simulink library "myLibrary"  (R2023a)
settings: Solver=VariableStepAuto  StartTime=0.0  StopTime=10.0  RelTol=1e-3
undefined symbols (not defined in the file): Cac_n1, ctrl1, Da, Discrete, dtha, ee_sli_rtmsupport, FA, gcbh, Ha, Ini, init_line, init_load, init_SG, init_TH, init_trafo, init_VSC, initMachineBlocks, Ka, Lf, Llkd_pu, Llkq1_pu, NET, P, plots_step, q0, Rac_n1, Radd, Rkd_pu, Rkq1_pu, Rload_add, sim_config, spsSteamTurbineModel, T_global, T_load, T_NET, T_SG, T_TH, T_trafo, T_VSC, Ts, tstep, V1
libraries: spsSeriesRLCBranchLib x57, spsParallelRLCBranchLib x39, eeGeneralControl x38, spsCurrentMeasurementLib x20, spsFirstOrderFilterLib x16, spsVoltageMeasurementLib x14, spsControlledVoltageSourceLib x12, $bdroot x9, dspsigops x6, spsThreePhaseVIMeasurementLib x5, spsPLL3phLib x4, spsThreePhaseBreakerLib x3
(part 2 of 7)

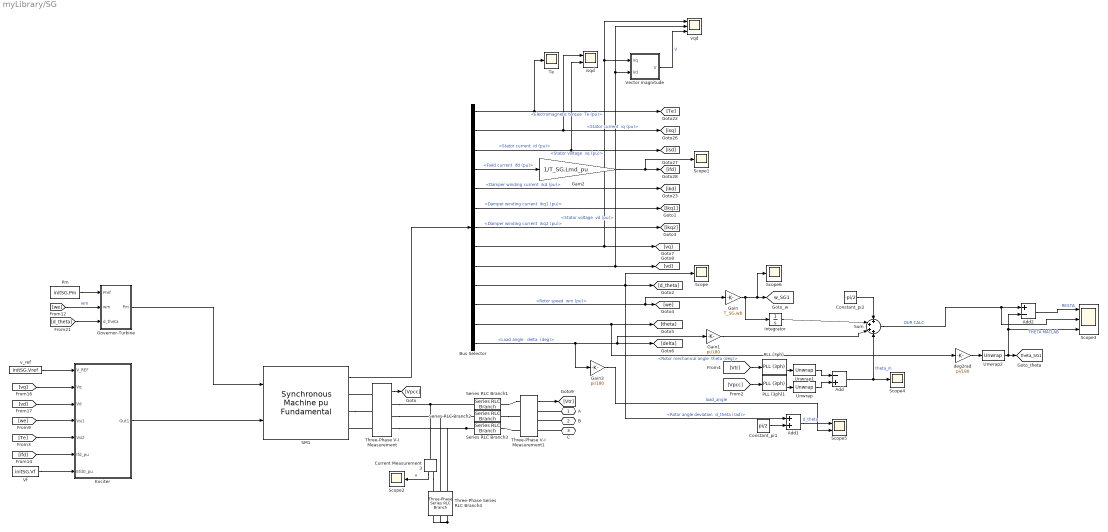
== system myLibrary/SG ==
  Add : Sum  Inputs=-+
  Add1 : Sum
  Add2 : Sum  Inputs=+-
  Bus Selector : BusSelector  OutputSignals="Mechanical.Electromagnetic torque  Te (pu),dq0 components.Stator current  iq (pu),dq0 components.Stator current  id (pu),dq0 components.Field current  ifd (pu),dq0 components.Damper winding current  ikd (pu),dq0 components.Damper winding current  ikq1 (pu),dq0 components.Damper winding current  ikq2 (pu),dq0 components.Stator voltage  vq (pu),dq0 components.Stator voltage  vd (pu),Mechanical.Rotor angle deviation  d_theta (rad),Mechanical.Rotor speed  wm (pu),Mechanical.Rotor mechanical angle  theta (deg),Load angle   delta  (deg)"
  Constant_pi1 : Constant  Value=pi/2
  Constant_pi2 : Constant  Value=-pi/2
  Current Measurement3 : spsCurrentMeasurementLib/Current Measurement  PhasorSimulation=off  OutputType=Complex  PSBequivalent=0
  Exciter : Subsystem
  Gain : Gain  Gain=T_SG.wb
  Gain1 : Gain  Gain=pi/180
  Gain2 : Gain  Gain=1/T_SG.Lmd_pu
  Gain3 : Gain  Gain=pi/180
  Governor-Turbine : Subsystem
  Integrator : Integrator
  PLL (3ph) : spsPLL3phLib/PLL (3ph)  Fmin=45  Par_Init=[0, 50]  ParK=[180, 3200, 1]  TcD=1e-4  MaxRateChangeFreq=12  FilterCutOffFreq=25  Ts=0  AGC=on
  PLL (3ph)1 : spsPLL3phLib/PLL (3ph)  Fmin=45  Par_Init=[initSG.theta_in, 50]  ParK=[180, 3200, 1]  TcD=1e-4  MaxRateChangeFreq=12  FilterCutOffFreq=25  Ts=0  AGC=on
  Pm : Constant  Value=initSG.Pm
  SM1 : spsSynchronousMachinepuFundamentalLib/Synchronous Machine pu Fundamental  PresetModel=No  MechanicalLoad=Mechanical power Pm  ShowDetailedParameters=on  RotorType=Round  Units=per unit fundamental parameters  MeasurementBus=off  NominalParameters=initMachineBlocks{SGnum,1}  Stator=initMachineBlocks{SGnum,2}  Field=initMachineBlocks{SGnum,3}  Dampers2=initMachineBlocks{SGnum,4}  Dampers1="[ Rkd_pu   Llkd_pu  Rkq1_pu  Llkq1_pu]"  Mechanical=initMachineBlocks{SGnum,5}  PolePairs=1  InitialConditions=initMachineBlocks{SGnum,6}  SetSaturation=off  Saturation=[0.6404,0.7127,0.8441,0.9214,0.9956,1.082,1.19,1.316,1.457;0.7,0.7698,0.8872,0.9466,0.9969,1.046,1.1,1.151,1.201]  LoadFlowParameters=[1 5.55 0 0 0]  TsPowergui=0  TsBlock=-1  IterativeModel=Trapezoidal non iterative  IterativeDiscreteModel=Trapezoidal non iterative  BusType=PV  Pref=5.55  Qref=0  Qmin=-Inf  Qmax=Inf  PLF=0  QLF=0
  Scope{,1..2,4,6} (5 alike) : Scope
  Scope3 : Scope  NumInputPorts=3
  Scope5 : Scope  NumInputPorts=2
  Series RLC Branch1 : spsSeriesRLCBranchLib/Series RLC Branch  LConnTagsString=__new0  RConnTagsString=__new0  BranchType=RL  Resistance=T_SG.Rtr*T_SG.Zbpu_l2g  Inductance=T_SG.Ltr*T_SG.Zbpu_l2g  SetiL0=off  InitialCurrent=initSG.Itr  Capacitance=P.C  Setx0=on  InitialVoltage=P.C  Measurements=None
  Series RLC Branch2 : spsSeriesRLCBranchLib/Series RLC Branch  LConnTagsString=__new0  RConnTagsString=__new0  BranchType=RL  Resistance=T_SG.Rtr*T_global.Sb(T_global.Area == T_SG.Area)/T_SG.Sb  Inductance=T_SG.Ltr*T_global.Sb(T_global.Area == T_SG.Area)/T_SG.Sb  SetiL0=off  InitialCurrent=initSG.Itr  Capacitance=P.C  Setx0=on  InitialVoltage=P.C  Measurements=None
  Series RLC Branch3 : spsSeriesRLCBranchLib/Series RLC Branch  LConnTagsString=__new0  RConnTagsString=__new0  BranchType=RL  Resistance=T_SG.Rtr*T_global.Sb(T_global.Area == T_SG.Area)/T_SG.Sb  Inductance=T_SG.Ltr*T_global.Sb(T_global.Area == T_SG.Area)/T_SG.Sb  SetiL0=off  InitialCurrent=initSG.Itr  Capacitance=P.C  Setx0=on  InitialVoltage=P.C  Measurements=None
  Sum : Sum  Inputs=++++
  Te : Scope
  Three-Phase Series RLC Branch4 : spsThreePhaseSeriesRLCBranchLib/Three-Phase Series RLC Branch  LConnTagsString=A|B|C  RConnTagsString=A|B|C  BranchType=R  Resistance=T_SG.Rsnb*T_SG.Zbpu_l2g  Inductance=NET.L1_2/2  Capacitance=1/0.0528/(2*pi*50)  Measurements=None
  Three-Phase V-I Measurement : spsThreePhaseVIMeasurementLib/Three-Phase V-I Measurement  VoltageMeasurement=phase-to-phase  SetLabelV=off  LabelV=Vpcc  Vpu=off  VpuLL=off  CurrentMeasurement=no  SetLabelI=off  LabelI=Iabc  Ipu=off  Pbase=100e6  Vbase=500e3  OutputType=Complex  PhasorSimulation=off  PSBequivalent=0
  Three-Phase V-I Measurement1 : spsThreePhaseVIMeasurementLib/Three-Phase V-I Measurement  VoltageMeasurement=phase-to-phase  SetLabelV=off  LabelV=Vtr  Vpu=off  VpuLL=off  CurrentMeasurement=no  SetLabelI=off  LabelI=Iabc  Ipu=off  Pbase=100e6  Vbase=500e3  OutputType=Complex  PhasorSimulation=off  PSBequivalent=0
  Unwrap : dspsigops/Unwrap  tol=pi  InputProcessing=Columns as channels (frame based)  running=off
  Unwrap1 : dspsigops/Unwrap  tol=pi  InputProcessing=Columns as channels (frame based)  running=off
  Unwrap2 : dspsigops/Unwrap  tol=pi  InputProcessing=Columns as channels (frame based)  running=off
  "Vector magnitude " : Subsystem
  Vf : Constant  Value=initSG.Vf
  deg2rad : Gain  Gain=pi/180
  isqd : Scope  NumInputPorts=2
  v_ref : Constant  Value=initSG.Vref
  vqd : Scope  NumInputPorts=3
  A : PMIOPort  Side=Right
  B : PMIOPort  Port=2  Side=Right
  C : PMIOPort  Port=3  Side=Right
  tag scope: theta_SG1=global, w_SG1=global
  wires:
  Three-Phase V-I Measurement1/1 -> [Vtr]
  Three-Phase V-I Measurement/1 -> [Vpcc]
  Bus Selector/10 -> [d_theta], Add1/1, Scope/1  "<Rotor angle deviation  d_theta (rad)>"
  Bus Selector/7 -> [ikq2]  "<Damper winding current  ikq2 (pu)>"
  [Vtr] -> PLL (3ph)/1
  Gain2/1 -> Scope1/1, [ifd]
  Bus Selector/5 -> [ikd]  "<Damper winding current  ikd (pu)>"
  Bus Selector/3 -> isqd/2, [isd]  "<Stator current  id (pu)>"
  Bus Selector/11 -> [we], Gain/1  "<Rotor speed  wm (pu)>"
  Bus Selector/6 -> [ikq1]  "<Damper winding current  ikq1 (pu)>"
  [Vpcc] -> PLL (3ph)1/1
  Bus Selector/4 -> Gain2/1  "<Field current  ifd (pu)>"
  Bus Selector/8 -> "Vector magnitude "/1(Vq), vqd/1, [vq]  "<Stator voltage  vq (pu)>"
  Bus Selector/1 -> Te/1, [Te]  "<Electromagnetic torque  Te (pu)>"
  Bus Selector/9 -> "Vector magnitude "/2(Vd), vqd/2, [vd]  "<Stator voltage  vd (pu)>"
  Gain/1 -> Scope6/1, [w_SG1], Integrator/1
  Current Measurement3/1 -> Scope2/1  "a"
  "Vector magnitude "/1(V) -> vqd/3  "V"
  Unwrap1/1 -> Add/1
  SM1/1 -> Bus Selector/1
  Bus Selector/13 -> [delta], Gain1/1, Gain3/1  "<Load angle   delta  (deg)>"
  Bus Selector/12 -> deg2rad/1, [theta]  "<Rotor mechanical angle  theta (deg)>"
  Bus Selector/2 -> isqd/1, [isq]  "<Stator current  iq (pu)>"
  Add/1 -> Scope4/1, Sum/4  "theta_in"
  Integrator/1 -> Sum/2
  PLL (3ph)1/2 -> Unwrap/1
  PLL (3ph)/2 -> Unwrap1/1
  Unwrap/1 -> Add/2
  Constant_pi1/1 -> Add1/2
  Add1/1 -> Scope5/1  "d_theta"
  Gain3/1 -> Scope5/2  "load_angle"
  Gain1/1 -> Sum/3
  Constant_pi2/1 -> Sum/1
  Governor-Turbine/1(Pm) -> SM1/1
  [we] -> Governor-Turbine/2(wm)  "wm"
  Pm/1 -> Governor-Turbine/1(Pref)
  [d_theta] -> Governor-Turbine/3(d_theta)
  deg2rad/1 -> Unwrap2/1
  Unwrap2/1 -> Add2/2, Scope3/3, [theta_SG1]  "THETA MATLAB"
  [we] -> Exciter/4(Vsi1)
  [vd] -> Exciter/3(Vd)
  [ifd] -> Exciter/6(Ifd_pu)
  [Te] -> Exciter/5(Vsi2)
  Vf/1 -> Exciter/7(Efd0_pu)
  v_ref/1 -> Exciter/1(V_REF)
  Exciter/1(Out1) -> SM1/2
  [vq] -> Exciter/2(Vq)
  Sum/1 -> Scope3/2, Add2/1  "OUR CALC"
  Add2/1 -> Scope3/1  "RESTA"
  connections:
  Three-Phase V-I Measurement/LConn3 -- SM1/RConn3
  SM1/RConn2 -- Three-Phase V-I Measurement/LConn2
  Three-Phase V-I Measurement/LConn1 -- SM1/RConn1
  B/RConn1 -- Three-Phase V-I Measurement1/RConn2
  Three-Phase V-I Measurement1/LConn3 -- Series RLC Branch3/RConn1
  Series RLC Branch1/RConn1 -- Three-Phase V-I Measurement1/LConn1
  Current Measurement3/RConn1 -- Three-Phase Series RLC Branch4/RConn1
  A/RConn1 -- Three-Phase V-I Measurement1/RConn1
  C/RConn1 -- Three-Phase V-I Measurement1/RConn3
  Series RLC Branch2/RConn1 -- Three-Phase V-I Measurement1/LConn2
  Three-Phase V-I Measurement/RConn1 -- Series RLC Branch1/LConn1 -- Current Measurement3/LConn1
  Series RLC Branch3/LConn1 -- Three-Phase V-I Measurement/RConn3 -- Three-Phase Series RLC Branch4/RConn3
  Three-Phase Series RLC Branch4/LConn3 -- Three-Phase Series RLC Branch4/LConn2 -- Three-Phase Series RLC Branch4/LConn1
  Series RLC Branch2/LConn1 -- Three-Phase V-I Measurement/RConn2 -- Three-Phase Series RLC Branch4/RConn2

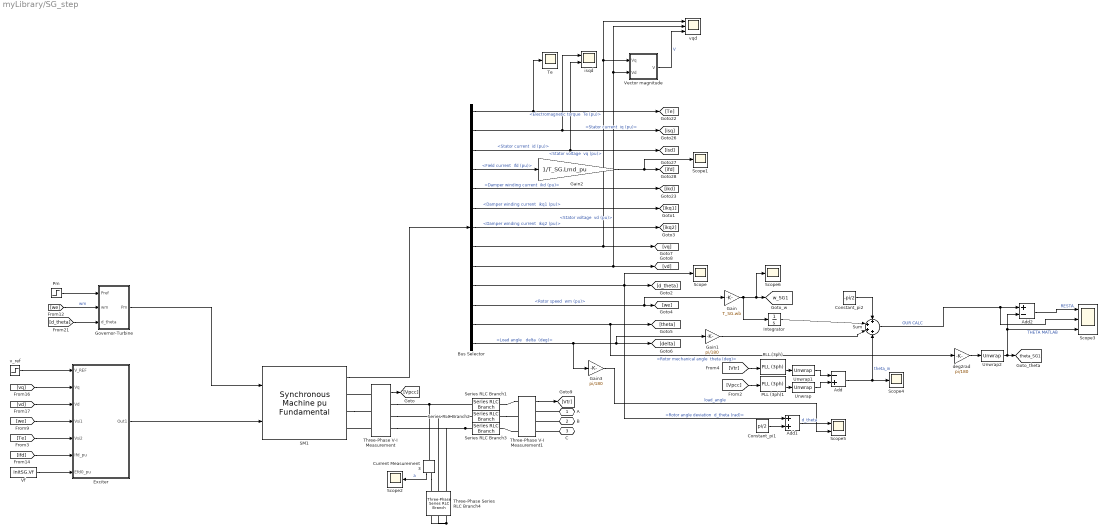
== system myLibrary/SG_step ==
  Add : Sum  Inputs=-+
  Add1 : Sum
  Add2 : Sum  Inputs=+-
  Bus Selector : BusSelector  OutputSignals="Mechanical.Electromagnetic torque  Te (pu),dq0 components.Stator current  iq (pu),dq0 components.Stator current  id (pu),dq0 components.Field current  ifd (pu),dq0 components.Damper winding current  ikd (pu),dq0 components.Damper winding current  ikq1 (pu),dq0 components.Damper winding current  ikq2 (pu),dq0 components.Stator voltage  vq (pu),dq0 components.Stator voltage  vd (pu),Mechanical.Rotor angle deviation  d_theta (rad),Mechanical.Rotor speed  wm (pu),Mechanical.Rotor mechanical angle  theta (deg),Load angle   delta  (deg)"
  Constant_pi1 : Constant  Value=pi/2
  Constant_pi2 : Constant  Value=-pi/2
  Current Measurement3 : spsCurrentMeasurementLib/Current Measurement  PhasorSimulation=off  OutputType=Complex  PSBequivalent=0
  Exciter : Subsystem
  Gain : Gain  Gain=T_SG.wb
  Gain1 : Gain  Gain=pi/180
  Gain2 : Gain  Gain=1/T_SG.Lmd_pu
  Gain3 : Gain  Gain=pi/180
  Governor-Turbine : Subsystem
  Integrator : Integrator
  PLL (3ph) : spsPLL3phLib/PLL (3ph)  Fmin=45  Par_Init=[0, 50]  ParK=[180, 3200, 1]  TcD=1e-4  MaxRateChangeFreq=12  FilterCutOffFreq=25  Ts=0  AGC=on
  PLL (3ph)1 : spsPLL3phLib/PLL (3ph)  Fmin=45  Par_Init=[initSG.theta_in, 50]  ParK=[180, 3200, 1]  TcD=1e-4  MaxRateChangeFreq=12  FilterCutOffFreq=25  Ts=0  AGC=on
  Pm : Step  Time=tstep_P  Before=initSG.Pm  After=initSG.Pm*(1+sim_config.DR)  SampleTime=1e-4
  SM1 : spsSynchronousMachinepuFundamentalLib/Synchronous Machine pu Fundamental  PresetModel=No  MechanicalLoad=Mechanical power Pm  ShowDetailedParameters=on  RotorType=Round  Units=per unit fundamental parameters  MeasurementBus=off  NominalParameters=initMachineBlocks{SGnum,1}  Stator=initMachineBlocks{SGnum,2}  Field=initMachineBlocks{SGnum,3}  Dampers2=initMachineBlocks{SGnum,4}  Dampers1="[ Rkd_pu   Llkd_pu  Rkq1_pu  Llkq1_pu]"  Mechanical=initMachineBlocks{SGnum,5}  PolePairs=1  InitialConditions=initMachineBlocks{SGnum,6}  SetSaturation=off  Saturation=[0.6404,0.7127,0.8441,0.9214,0.9956,1.082,1.19,1.316,1.457;0.7,0.7698,0.8872,0.9466,0.9969,1.046,1.1,1.151,1.201]  LoadFlowParameters=[1 5.55 0 0 0]  TsPowergui=0  TsBlock=-1  IterativeModel=Trapezoidal non iterative  IterativeDiscreteModel=Trapezoidal non iterative  BusType=PV  Pref=5.55  Qref=0  Qmin=-Inf  Qmax=Inf  PLF=0  QLF=0
  Scope{,1..2,4,6} (5 alike) : Scope
  Scope3 : Scope  NumInputPorts=3
  Scope5 : Scope  NumInputPorts=2
  Series RLC Branch1 : spsSeriesRLCBranchLib/Series RLC Branch  LConnTagsString=__new0  RConnTagsString=__new0  BranchType=RL  Resistance=T_SG.Rtr*T_SG.Zbpu_l2g  Inductance=T_SG.Ltr*T_SG.Zbpu_l2g  SetiL0=off  InitialCurrent=initSG.Itr  Capacitance=P.C  Setx0=on  InitialVoltage=P.C  Measurements=None
  Series RLC Branch2 : spsSeriesRLCBranchLib/Series RLC Branch  LConnTagsString=__new0  RConnTagsString=__new0  BranchType=RL  Resistance=T_SG.Rtr*T_global.Sb(T_global.Area == T_SG.Area)/T_SG.Sb  Inductance=T_SG.Ltr*T_global.Sb(T_global.Area == T_SG.Area)/T_SG.Sb  SetiL0=off  InitialCurrent=initSG.Itr  Capacitance=P.C  Setx0=on  InitialVoltage=P.C  Measurements=None
  Series RLC Branch3 : spsSeriesRLCBranchLib/Series RLC Branch  LConnTagsString=__new0  RConnTagsString=__new0  BranchType=RL  Resistance=T_SG.Rtr*T_global.Sb(T_global.Area == T_SG.Area)/T_SG.Sb  Inductance=T_SG.Ltr*T_global.Sb(T_global.Area == T_SG.Area)/T_SG.Sb  SetiL0=off  InitialCurrent=initSG.Itr  Capacitance=P.C  Setx0=on  InitialVoltage=P.C  Measurements=None
  Sum : Sum  Inputs=++++
  Te : Scope
  Three-Phase Series RLC Branch4 : spsThreePhaseSeriesRLCBranchLib/Three-Phase Series RLC Branch  LConnTagsString=A|B|C  RConnTagsString=A|B|C  BranchType=R  Resistance=T_SG.Rsnb*T_SG.Zbpu_l2g  Inductance=NET.L1_2/2  Capacitance=1/0.0528/(2*pi*50)  Measurements=None
  Three-Phase V-I Measurement : spsThreePhaseVIMeasurementLib/Three-Phase V-I Measurement  VoltageMeasurement=phase-to-phase  SetLabelV=off  LabelV=Vpcc  Vpu=off  VpuLL=off  CurrentMeasurement=no  SetLabelI=off  LabelI=Iabc  Ipu=off  Pbase=100e6  Vbase=500e3  OutputType=Complex  PhasorSimulation=off  PSBequivalent=0
  Three-Phase V-I Measurement1 : spsThreePhaseVIMeasurementLib/Three-Phase V-I Measurement  VoltageMeasurement=phase-to-phase  SetLabelV=off  LabelV=Vtr  Vpu=off  VpuLL=off  CurrentMeasurement=no  SetLabelI=off  LabelI=Iabc  Ipu=off  Pbase=100e6  Vbase=500e3  OutputType=Complex  PhasorSimulation=off  PSBequivalent=0
  Unwrap : dspsigops/Unwrap  tol=pi  InputProcessing=Columns as channels (frame based)  running=off
  Unwrap1 : dspsigops/Unwrap  tol=pi  InputProcessing=Columns as channels (frame based)  running=off
  Unwrap2 : dspsigops/Unwrap  tol=pi  InputProcessing=Columns as channels (frame based)  running=off
  "Vector magnitude " : Subsystem
  Vf : Constant  Value=initSG.Vf
  deg2rad : Gain  Gain=pi/180
  isqd : Scope  NumInputPorts=2
  v_ref : Step  Time=tstep_V  Before=initSG.Vref  After=initSG.Vref*(1+sim_config.DR)  SampleTime=1e-4
  vqd : Scope  NumInputPorts=3
  A : PMIOPort  Side=Right
  B : PMIOPort  Port=2  Side=Right
  C : PMIOPort  Port=3  Side=Right
  tag scope: theta_SG1=global, w_SG1=global
  wires:
  Three-Phase V-I Measurement1/1 -> [Vtr]
  Three-Phase V-I Measurement/1 -> [Vpcc]
  Bus Selector/10 -> [d_theta], Add1/1, Scope/1  "<Rotor angle deviation  d_theta (rad)>"
  Bus Selector/7 -> [ikq2]  "<Damper winding current  ikq2 (pu)>"
  [Vtr] -> PLL (3ph)/1
  Gain2/1 -> Scope1/1, [ifd]
  Bus Selector/5 -> [ikd]  "<Damper winding current  ikd (pu)>"
  Bus Selector/3 -> isqd/2, [isd]  "<Stator current  id (pu)>"
  Bus Selector/11 -> [we], Gain/1  "<Rotor speed  wm (pu)>"
  Bus Selector/6 -> [ikq1]  "<Damper winding current  ikq1 (pu)>"
  [Vpcc] -> PLL (3ph)1/1
  Bus Selector/4 -> Gain2/1  "<Field current  ifd (pu)>"
  Bus Selector/8 -> "Vector magnitude "/1(Vq), vqd/1, [vq]  "<Stator voltage  vq (pu)>"
  Bus Selector/1 -> Te/1, [Te]  "<Electromagnetic torque  Te (pu)>"
  Bus Selector/9 -> "Vector magnitude "/2(Vd), vqd/2, [vd]  "<Stator voltage  vd (pu)>"
  Gain/1 -> Scope6/1, [w_SG1], Integrator/1
  Current Measurement3/1 -> Scope2/1  "a"
  "Vector magnitude "/1(V) -> vqd/3  "V"
  Unwrap1/1 -> Add/1
  SM1/1 -> Bus Selector/1
  Bus Selector/13 -> [delta], Gain1/1, Gain3/1  "<Load angle   delta  (deg)>"
  Bus Selector/12 -> deg2rad/1, [theta]  "<Rotor mechanical angle  theta (deg)>"
  Bus Selector/2 -> isqd/1, [isq]  "<Stator current  iq (pu)>"
  Add/1 -> Scope4/1, Sum/4  "theta_in"
  Integrator/1 -> Sum/2
  PLL (3ph)1/2 -> Unwrap/1
  PLL (3ph)/2 -> Unwrap1/1
  Unwrap/1 -> Add/2
  Constant_pi1/1 -> Add1/2
  Add1/1 -> Scope5/1  "d_theta"
  Gain3/1 -> Scope5/2  "load_angle"
  Gain1/1 -> Sum/3
  Constant_pi2/1 -> Sum/1
  Governor-Turbine/1(Pm) -> SM1/1
  [we] -> Governor-Turbine/2(wm)  "wm"
  Pm/1 -> Governor-Turbine/1(Pref)
  [d_theta] -> Governor-Turbine/3(d_theta)
  deg2rad/1 -> Unwrap2/1
  Unwrap2/1 -> Add2/2, Scope3/3, [theta_SG1]  "THETA MATLAB"
  [we] -> Exciter/4(Vsi1)
  [vd] -> Exciter/3(Vd)
  [ifd] -> Exciter/6(Ifd_pu)
  [Te] -> Exciter/5(Vsi2)
  Vf/1 -> Exciter/7(Efd0_pu)
  v_ref/1 -> Exciter/1(V_REF)
  Exciter/1(Out1) -> SM1/2
  [vq] -> Exciter/2(Vq)
  Sum/1 -> Scope3/2, Add2/1  "OUR CALC"
  Add2/1 -> Scope3/1  "RESTA"
  connections:
  Three-Phase V-I Measurement/LConn3 -- SM1/RConn3
  SM1/RConn2 -- Three-Phase V-I Measurement/LConn2
  Three-Phase V-I Measurement/LConn1 -- SM1/RConn1
  B/RConn1 -- Three-Phase V-I Measurement1/RConn2
  Three-Phase V-I Measurement1/LConn3 -- Series RLC Branch3/RConn1
  Series RLC Branch1/RConn1 -- Three-Phase V-I Measurement1/LConn1
  Current Measurement3/RConn1 -- Three-Phase Series RLC Branch4/RConn1
  A/RConn1 -- Three-Phase V-I Measurement1/RConn1
  C/RConn1 -- Three-Phase V-I Measurement1/RConn3
  Series RLC Branch2/RConn1 -- Three-Phase V-I Measurement1/LConn2
  Three-Phase V-I Measurement/RConn1 -- Series RLC Branch1/LConn1 -- Current Measurement3/LConn1
  Series RLC Branch3/LConn1 -- Three-Phase V-I Measurement/RConn3 -- Three-Phase Series RLC Branch4/RConn3
  Three-Phase Series RLC Branch4/LConn3 -- Three-Phase Series RLC Branch4/LConn2 -- Three-Phase Series RLC Branch4/LConn1
  Series RLC Branch2/LConn1 -- Three-Phase V-I Measurement/RConn2 -- Three-Phase Series RLC Branch4/RConn2

== system myLibrary/TH ==
  note: Grid Thevenin
  Series RLC Branch : spsSeriesRLCBranchLib/Series RLC Branch  LConnTagsString=__new0  RConnTagsString=__new0  BranchType=RL  Resistance=T.R  Inductance=T.L  SetiL0=off  InitialCurrent=ini.Itha  Capacitance=1e-6  Setx0=off  InitialVoltage=0  Measurements=None
  Series RLC Branch1 : spsSeriesRLCBranchLib/Series RLC Branch  LConnTagsString=__new0  RConnTagsString=__new0  BranchType=RL  Resistance=T.R  Inductance=T.L  SetiL0=on  InitialCurrent=ini.Ithb  Capacitance=1e-6  Setx0=off  InitialVoltage=0  Measurements=None
  Series RLC Branch2 : spsSeriesRLCBranchLib/Series RLC Branch  LConnTagsString=__new0  RConnTagsString=__new0  BranchType=RL  Resistance=T.R  Inductance=T.L  SetiL0=on  InitialCurrent=ini.Ithc  Capacitance=1e-6  Setx0=off  InitialVoltage=0  Measurements=None
  Three-Phase Source : spsThreePhaseSourceLib/Three-Phase Source  InternalConnection=Y  VoltagePhases=off  Voltage=ini.Vmag  PhaseAngle=ini.angle*180/pi  Voltage_phases=[25e3 25e3 25e3]/sqrt(3)  PhaseAngles_phases=[0 -120 +120]  Frequency="T_global{T_global.Area == T.Area,\"fb\"}"  NonIdealSource=off  SpecifyImpedance=off  Resistance=0.8929  Inductance=16.58e-3  ShortCircuitLevel=100e6  BaseVoltage=25e3  XRratio=7  BusType=swing  Pref=10e3  Qref=0  Prefabc=[10e3, 10e3, 10e3]  Qrefabc=[0, 0, 0]  Qmin=-inf  Qmax=inf
  A : PMIOPort  Side=Right
  B : PMIOPort  Port=2  Side=Right
  C : PMIOPort  Port=3  Side=Right
  connections:
  Series RLC Branch1/LConn1 -- Three-Phase Source/RConn2
  Series RLC Branch/LConn1 -- Three-Phase Source/RConn1
  A/RConn1 -- Series RLC Branch/RConn1
  B/RConn1 -- Series RLC Branch1/RConn1
  Series RLC Branch2/LConn1 -- Three-Phase Source/RConn3
  C/RConn1 -- Series RLC Branch2/RConn1

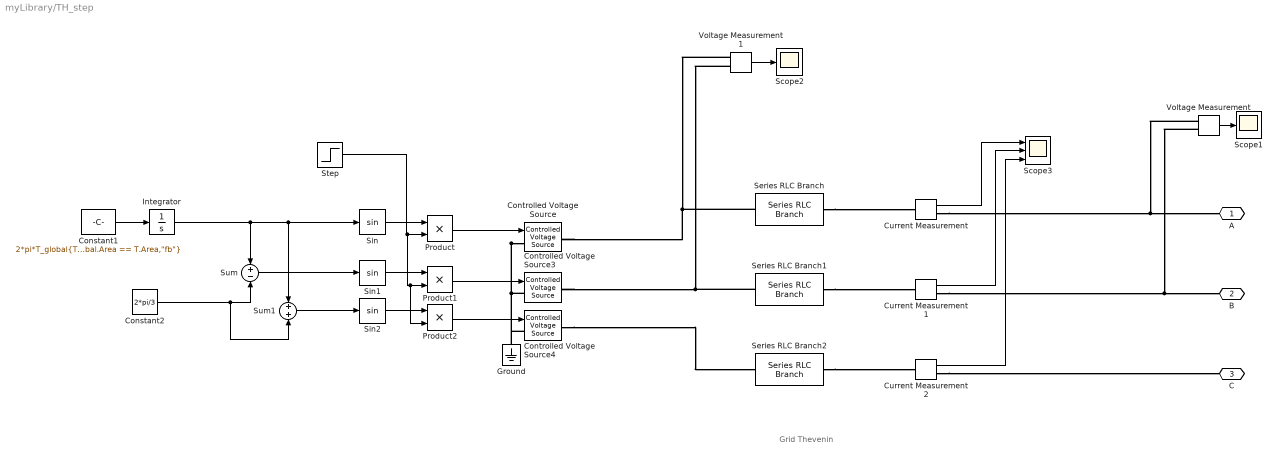
== system myLibrary/TH_step ==
  note: Grid Thevenin
  Constant1 : Constant  Value="2*pi*T_global{T_global.Area == T.Area,\"fb\"}"
  Constant2 : Constant  Value=2*pi/3
  Controlled Voltage Source : spsControlledVoltageSourceLib/Controlled Voltage Source  Initialize=on  Source_Type=AC  Amplitude=ini.Vmag/sqrt(3)*sqrt(2)  Phase=ini.angle*180/pi  Frequency=T_global.f_Hz  Measurements=None
  Controlled Voltage Source3 : spsControlledVoltageSourceLib/Controlled Voltage Source  Initialize=on  Source_Type=AC  Amplitude=ini.Vmag/sqrt(3)*sqrt(2)  Phase=ini.angle*180/pi-120  Frequency=T_global.f_Hz  Measurements=None
  Controlled Voltage Source4 : spsControlledVoltageSourceLib/Controlled Voltage Source  Initialize=on  Source_Type=AC  Amplitude=ini.Vmag/sqrt(3)*sqrt(2)  Phase=ini.angle*180/pi+120  Frequency=T_global.f_Hz  Measurements=None
  Current Measurement : spsCurrentMeasurementLib/Current Measurement  PhasorSimulation=off  OutputType=Complex  PSBequivalent=0
  Current Measurement1 : spsCurrentMeasurementLib/Current Measurement  PhasorSimulation=off  OutputType=Complex  PSBequivalent=0
  Current Measurement2 : spsCurrentMeasurementLib/Current Measurement  PhasorSimulation=off  OutputType=Complex  PSBequivalent=0
  Ground : spsGroundLib/Ground  LConnTagsString=a
  Integrator : Integrator  InitialCondition=ini.angle
  Product : Product
  Product1 : Product
  Product2 : Product
  Scope1 : Scope
  Scope2 : Scope
  Scope3 : Scope  NumInputPorts=3
  Series RLC Branch : spsSeriesRLCBranchLib/Series RLC Branch  LConnTagsString=__new0  RConnTagsString=__new0  BranchType=RL  Resistance=T.R  Inductance=T.L  SetiL0=on  InitialCurrent=ini.Itha  Capacitance=1e-6  Setx0=off  InitialVoltage=0  Measurements=None
  Series RLC Branch1 : spsSeriesRLCBranchLib/Series RLC Branch  LConnTagsString=__new0  RConnTagsString=__new0  BranchType=RL  Resistance=T.R  Inductance=T.L  SetiL0=on  InitialCurrent=ini.Ithb  Capacitance=1e-6  Setx0=off  InitialVoltage=0  Measurements=None
  Series RLC Branch2 : spsSeriesRLCBranchLib/Series RLC Branch  LConnTagsString=__new0  RConnTagsString=__new0  BranchType=RL  Resistance=T.R  Inductance=T.L  SetiL0=on  InitialCurrent=ini.Ithc  Capacitance=1e-6  Setx0=off  InitialVoltage=0  Measurements=None
  Sin : Trigonometry
  Sin1 : Trigonometry
  Sin2 : Trigonometry
  Step : Step  Time=tstep  Before=ini.Vmag/sqrt(3)*sqrt(2)  After=V1/sqrt(3)*sqrt(2)  SampleTime=1e-4
  Sum : Sum  Inputs=+-
  Sum1 : Sum
  Voltage Measurement : spsVoltageMeasurementLib/Voltage Measurement  PhasorSimulation=off  OutputType=Complex  PSBequivalent=0
  Voltage Measurement1 : spsVoltageMeasurementLib/Voltage Measurement  PhasorSimulation=off  OutputType=Complex  PSBequivalent=0
  A : PMIOPort  Side=Right
  B : PMIOPort  Port=2  Side=Right
  C : PMIOPort  Port=3  Side=Right
  wires:
  Current Measurement2/1 -> Scope3/3
  Current Measurement1/1 -> Scope3/2
  Current Measurement/1 -> Scope3/1
  Voltage Measurement1/1 -> Scope2/1
  Voltage Measurement/1 -> Scope1/1
  Sum1/1 -> Sin2/1
  Sin/1 -> Product/1
  Product1/1 -> Controlled Voltage Source3/1
  Product/1 -> Controlled Voltage Source/1
  Sum/1 -> Sin1/1
  Sin1/1 -> Product1/1
  Step/1 -> Product2/2, Product1/2, Product/2
  Sin2/1 -> Product2/1
  Product2/1 -> Controlled Voltage Source4/1
  Constant1/1 -> Integrator/1
  Constant2/1 -> Sum1/2, Sum/2
  Integrator/1 -> Sum/1, Sum1/1, Sin/1
  connections:
  Current Measurement2/RConn1 -- C/RConn1
  Voltage Measurement1/LConn2 -- Controlled Voltage Source3/RConn1 -- Series RLC Branch1/LConn1
  Voltage Measurement1/LConn1 -- Controlled Voltage Source/RConn1 -- Series RLC Branch/LConn1
  Current Measurement1/RConn1 -- B/RConn1 -- Voltage Measurement/LConn2
  Current Measurement/RConn1 -- A/RConn1 -- Voltage Measurement/LConn1
  Series RLC Branch/RConn1 -- Current Measurement/LConn1
  Series RLC Branch1/RConn1 -- Current Measurement1/LConn1
  Controlled Voltage Source4/RConn1 -- Series RLC Branch2/LConn1
  Series RLC Branch2/RConn1 -- Current Measurement2/LConn1
  Controlled Voltage Source/LConn1 -- Controlled Voltage Source4/LConn1 -- Ground/LConn1 -- Controlled Voltage Source3/LConn1

== system myLibrary/Trafo ==
  Series RLC Branch1 : spsSeriesRLCBranchLib/Series RLC Branch  LConnTagsString=__new0  RConnTagsString=__new0  BranchType=RL  Resistance=T.R  Inductance=T.L  SetiL0=on  InitialCurrent=ini.Ia  Capacitance=P.C  Setx0=on  InitialVoltage=P.C  Measurements=None
  Series RLC Branch2 : spsSeriesRLCBranchLib/Series RLC Branch  LConnTagsString=__new0  RConnTagsString=__new0  BranchType=RL  Resistance=T.R  Inductance=T.L  SetiL0=on  InitialCurrent=ini.Ib  Capacitance=P.C  Setx0=on  InitialVoltage=P.C  Measurements=None
  Series RLC Branch3 : spsSeriesRLCBranchLib/Series RLC Branch  LConnTagsString=__new0  RConnTagsString=__new0  BranchType=RL  Resistance=T.R  Inductance=T.L  SetiL0=on  InitialCurrent=ini.Ic  Capacitance=P.C  Setx0=on  InitialVoltage=P.C  Measurements=None
  A1 : PMIOPort  Side=Left
  B1 : PMIOPort  Port=2  Side=Left
  C1 : PMIOPort  Port=3  Side=Left
  A2 : PMIOPort  Port=4  Side=Right
  B2 : PMIOPort  Port=5  Side=Right
  C2 : PMIOPort  Port=6  Side=Right
  connections:
  Series RLC Branch1/RConn1 -- A2/RConn1
  Series RLC Branch2/RConn1 -- B2/RConn1
  Series RLC Branch3/RConn1 -- C2/RConn1
  Series RLC Branch2/LConn1 -- B1/RConn1
  Series RLC Branch1/LConn1 -- A1/RConn1
  Series RLC Branch3/LConn1 -- C1/RConn1

== system myLibrary/qd transform ==
  abc : Inport
  angle : Inport  Port=2
  Demux8 : Demux  Outputs=3
  qd0 Transformation : Subsystem
  q : Outport
  d : Outport  Port=2
  wires:
  qd0 Transformation/1(q) -> q/1  "q"
  Demux8/1 -> qd0 Transformation/1(a)
  qd0 Transformation/2(d) -> d/1  "d"
  Demux8/2 -> qd0 Transformation/2(b)
  abc/1 -> Demux8/1
  Demux8/3 -> qd0 Transformation/3(c)
  angle/1 -> qd0 Transformation/4(Angle)

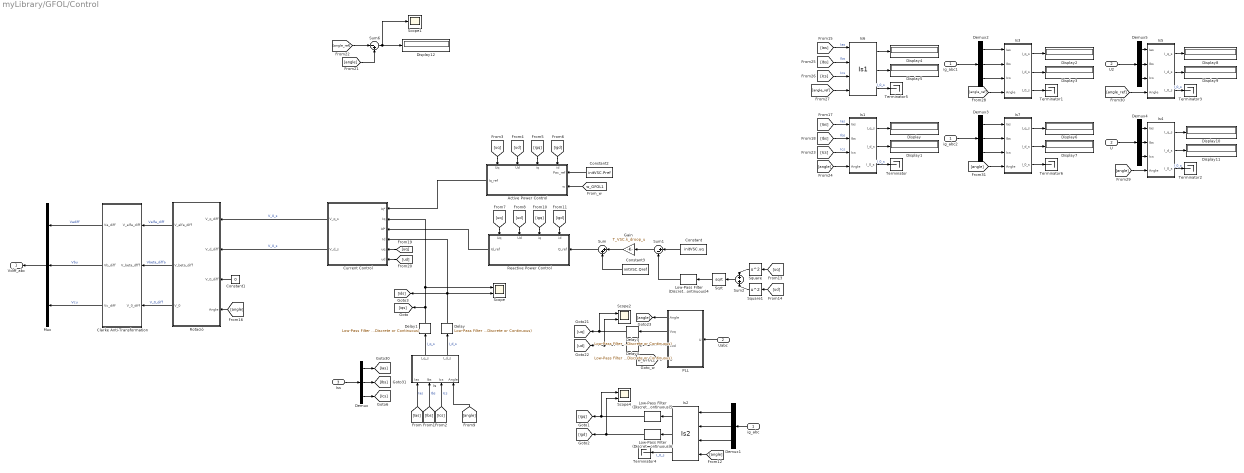
== system myLibrary/GFOL/Control ==
  ig_abc : Inport
  U : Inport  Port=2
  Iss : Inport  Port=3
  Active Power Control : Subsystem
      settings: PortSchema="{\"entries\":[{\"content\":{\"sides\":[{\"content\":{\"connectorIds\":[\"In1\",\"In2\"]},\"type\":\"ConnectorPlacement.EquallySpacedRectSide\",\"uuid\":\"78fe08fc-97ab-4d3f-ad1e-a4935a540f0d\"},{\"content\":{\"connectorIds\":[\"Out1\"],\"side\":\"RIGHT\"},\"type\":\"ConnectorPlacement.EquallySpacedRectSide\",\"uuid\":\"fec6fd50-7083-47ad-a120-ce0b4b3eb939\"},{\"content\":{\"connectorIds\":[\"In3\",\"In4\",\"In5\",\"In6\"],\"side\":\"TOP\"},\"type\":\"ConnectorPlacement.EquallySpacedRectSide\",\"uuid\":\"cab1bf13-1988-4815-ae0e-163353411583\"}]},\"type\":\"ConnectorPlacement.EquallySpacedConnector\",\"uuid\":\"1108cbfd-0203-4acc-b5d3-05af7402b6e2\"}],\"packageUris\":[\"http://schema.mathworks.com/mf0/Connector/R2020b\"],\"version\":\"1.0\"}"
  Clarke Anti-Transformation : Subsystem
  Constant : Constant  Value=initVSC.uq
  Constant1 : Constant  Value=0
  Constant2 : Constant  Value=initVSC.Pref
  Constant3 : Constant  Value=initVSC.Qref
  Current Control : Subsystem
  Delay : eeGeneralControl/Low-Pass Filter (Discrete or Continuous)  K=1  T=init_VSC.delay  B=inf  A=-inf  init_option=Specify as parameter  x0=initVSC.idiffd  Ts=0
  Delay1 : eeGeneralControl/Low-Pass Filter (Discrete or Continuous)  K=1  T=init_VSC.delay  B=inf  A=-inf  init_option=Specify as parameter  x0=initVSC.idiffq  Ts=0
  Delay3 : eeGeneralControl/Low-Pass Filter (Discrete or Continuous)  K=1  T=init_VSC.delay  B=inf  A=-inf  init_option=Specify as parameter  x0=initVSC.uq  Ts=0
  Delay4 : eeGeneralControl/Low-Pass Filter (Discrete or Continuous)  K=1  T=init_VSC.delay  B=inf  A=-inf  init_option=Specify as parameter  x0=initVSC.ud  Ts=0
  Demux{,1..5} (6 alike) : Demux  Outputs=3
  Display{,1..12} (13 alike) : Display
  Gain : Gain  Gain=T_VSC.k_droop_u
  Is : Subsystem
  Is1 : Subsystem
  Is2 : $bdroot/GFOR/Control/Is2  SystemSampleTime=-1  VariantActivationTime=update diagram  Latency=0  AutoFrameSizeCalculation=off
  Is3 : Subsystem
  Is4 : Subsystem
  Is5 : Subsystem
  Is6 : $bdroot/GFOL/Control/Is1  SystemSampleTime=-1  VariantActivationTime=update diagram  Latency=0  AutoFrameSizeCalculation=off
  Is7 : Subsystem
  Low-Pass Filter (Discrete or Continuous)4 : eeGeneralControl/Low-Pass Filter (Discrete or Continuous)  K=1  T=T_VSC.tau_droop_u  B=inf  A=-inf  init_option=Specify as parameter  x0=initVSC.uq  Ts=-1
  Low-Pass Filter (Discrete or Continuous)5 : eeGeneralControl/Low-Pass Filter (Discrete or Continuous)  K=1  T=init_VSC.delay  B=inf  A=-inf  init_option=Specify as parameter  x0=initVSC.igq  Ts=0
  Low-Pass Filter (Discrete or Continuous)6 : eeGeneralControl/Low-Pass Filter (Discrete or Continuous)  K=1  T=init_VSC.delay  B=inf  A=-inf  init_option=Specify as parameter  x0=initVSC.igd  Ts=0
  Mux : Mux  Inputs=3
  PLL : Subsystem
  Reactive Power Control : Subsystem
      settings: PortSchema="{\"entries\":[{\"content\":{\"sides\":[{\"content\":{\"connectorIds\":[\"In1\"]},\"type\":\"ConnectorPlacement.EquallySpacedRectSide\",\"uuid\":\"78fe08fc-97ab-4d3f-ad1e-a4935a540f0d\"},{\"content\":{\"connectorIds\":[\"Out1\"],\"side\":\"RIGHT\"},\"type\":\"ConnectorPlacement.EquallySpacedRectSide\",\"uuid\":\"fec6fd50-7083-47ad-a120-ce0b4b3eb939\"},{\"content\":{\"connectorIds\":[\"In2\",\"In3\",\"In4\",\"In5\"],\"side\":\"TOP\"},\"type\":\"ConnectorPlacement.EquallySpacedRectSide\",\"uuid\":\"cab1bf13-1988-4815-ae0e-163353411583\"}]},\"type\":\"ConnectorPlacement.EquallySpacedConnector\",\"uuid\":\"1108cbfd-0203-4acc-b5d3-05af7402b6e2\"}],\"packageUris\":[\"http://schema.mathworks.com/mf0/Connector/R2020b\"],\"version\":\"1.0\"}"
  Rotació : Subsystem
  Scope : Scope  NumInputPorts=2
  Scope1 : Scope
  Scope2 : Scope  NumInputPorts=2
  Scope4 : Scope  NumInputPorts=2
  Sqrt : Sqrt
  Square : Math  Operator=square
  Square1 : Math  Operator=square
  Sum : Sum  Inputs=|++
  Sum1 : Sum  Inputs=|+-
  Sum2 : Sum
  Sum6 : Sum  Inputs=|-+
  Terminator{,1..6} (7 alike) : Terminator
  U2 : InportShadow  Port=2
  Uabc : InportShadow  Port=2
  ig_abc1 : InportShadow
  ig_abc2 : InportShadow
  Vdiff_abc : Outport
  tag scope: w_GFOL1=global
  wires:
  Demux1/2 -> Is2/2
  Is2/1 -> Low-Pass Filter (Discrete or Continuous)5/1
  [angle] -> Is2/4
  Is2/2 -> Low-Pass Filter (Discrete or Continuous)6/1
  Is2/3 -> Terminator4/1  "I_0_s"
  Low-Pass Filter (Discrete or Continuous)6/1 -> Scope4/2, [igd]
  ig_abc/1 -> Demux1/1
  Demux1/3 -> Is2/3
  Demux1/1 -> Is2/1
  Low-Pass Filter (Discrete or Continuous)5/1 -> [igq], Scope4/1
  Sqrt/1 -> Low-Pass Filter (Discrete or Continuous)4/1
  Delay4/1 -> [ud], Scope2/2
  Delay3/1 -> Scope2/1, [uq]
  Constant/1 -> Sum1/1
  Low-Pass Filter (Discrete or Continuous)4/1 -> Sum1/2
  Sum2/1 -> Sqrt/1
  Square1/1 -> Sum2/2
  Square/1 -> Sum2/1
  [ud] -> Square1/1
  [uq] -> Square/1
  Sum1/1 -> Gain/1
  Gain/1 -> Sum/1
  Constant3/1 -> Sum/2
  Sum/1 -> Reactive Power Control/1(Q_ref)
  [w_GFOL1] -> Active Power Control/2(w)
  PLL/4(w) -> [w_GFOL1]
  Is/2(I_d_s) -> Delay/1  "I_d_s"
  Is/1(I_q_s) -> Delay1/1  "I_q_s"
  [Ias] -> Is/1(Ias)  "Ias"
  [Ics] -> Is/3(Ics)  "Ics"
  [Ibs] -> Is/2(Ibs)  "Ibs"
  PLL/1(Angle) -> [angle]
  Uabc/1 -> PLL/1(U)
  Demux/1 -> [Ias]
  Demux/2 -> [Ibs]
  Demux/3 -> [Ics]
  Iss/1 -> Demux/1
  [angle] -> Is/4(Angle)
  [angle] -> Rotació/4(Angle)
  Current Control/1(V_q_s) -> Rotació/1(V_q_diff)  "V_0_s"
  Current Control/2(V_d_s) -> Rotació/2(V_d_diff)  "V_0_s"
  [uq] -> Current Control/5(uq)
  [ud] -> Current Control/6(ud)
  [angle] -> Sum6/2
  Sum6/1 -> Scope1/1, Display12/1
  [angle_ref] -> Sum6/1
  [Ias] -> Is1/1(Ias)  "Ias"
  [Ibs] -> Is1/2(Ibs)  "Ibs"
  [Ics] -> Is1/3(Ics)  "Ics"
  [angle] -> Is1/4(Angle)
  [angle_ref] -> Is3/4(Angle)
  U/1 -> Demux4/1
  Demux4/1 -> Is4/1(Ias)
  Demux4/2 -> Is4/2(Ibs)
  Demux4/3 -> Is4/3(Ics)
  [angle] -> Is4/4(Angle)
  [angle_ref] -> Is5/4(Angle)
  Demux5/3 -> Is5/3(Ics)
  Demux5/2 -> Is5/2(Ibs)
  Demux5/1 -> Is5/1(Ias)
  U2/1 -> Demux5/1
  Is1/1(I_q_s) -> Display/1
  Is1/2(I_d_s) -> Display1/1
  Is3/1(I_q_s) -> Display2/1
  Is3/2(I_d_s) -> Display3/1
  Is4/1(I_q_s) -> Display10/1
  Is4/2(I_d_s) -> Display11/1
  Is5/1(I_q_s) -> Display8/1
  Is5/2(I_d_s) -> Display9/1
  Is1/3(I_0_s) -> Terminator/1  "I_0_s"
  Is3/3(I_0_s) -> Terminator1/1
  Is4/3(I_0_s) -> Terminator2/1  "I_0_s"
  Is5/3(I_0_s) -> Terminator3/1  "I_0_s"
  Rotació/1(V_alfa_diff) -> Clarke Anti-Transformation/1(V_alfa_diff)  "Valfa_diff"
  Rotació/2(V_beta_diff) -> Clarke Anti-Transformation/2(V_beta_dfff)  "Vbeta_diffa"
  Clarke Anti-Transformation/1(Va_diff) -> Mux/1  "Vadiff"
  Rotació/3(V_0) -> Clarke Anti-Transformation/3(V_0_diff)  "V_0_diff"
  Clarke Anti-Transformation/3(Vc_diff) -> Mux/3  "Vcu"
  Clarke Anti-Transformation/2(Vb_diff) -> Mux/2  "Vbu"
  Mux/1 -> Vdiff_abc/1
  [uq] -> Active Power Control/6(Uq)
  [ud] -> Active Power Control/5(Ud)
  Active Power Control/1(Iq_ref) -> Current Control/1(Iq*)
  Delay/1 -> Scope/2, Current Control/4(Id), [ids]
  Delay1/1 -> Current Control/2(Iq), Scope/1, [iqs]
  Constant1/1 -> Rotació/3(V_0_diff)
  PLL/2(Vzq) -> Delay3/1
  PLL/3(Vzd) -> Delay4/1
  [igq] -> Active Power Control/4(iq)
  [igd] -> Active Power Control/3(id)
  Constant2/1 -> Active Power Control/1(Pac_ref)
  [igd] -> Reactive Power Control/2(id)
  [igq] -> Reactive Power Control/3(iq)
  [ud] -> Reactive Power Control/4(Ud)
  [uq] -> Reactive Power Control/5(Uq)
  Reactive Power Control/1(Id_ref) -> Current Control/3(Id*)
  Demux2/1 -> Is3/1(Ias)
  Demux2/2 -> Is3/2(Ibs)
  Demux2/3 -> Is3/3(Ics)
  ig_abc1/1 -> Demux2/1
  Is6/3 -> Terminator5/1  "I_0_s"
  Is6/2 -> Display5/1
  Is6/1 -> Display4/1
  [angle_ref] -> Is6/4
  [Ics] -> Is6/3  "Ics"
  [Ibs] -> Is6/2  "Ibs"
  [Ias] -> Is6/1  "Ias"
  ig_abc2/1 -> Demux3/1
  Demux3/3 -> Is7/3(Ics)
  Demux3/2 -> Is7/2(Ibs)
  Demux3/1 -> Is7/1(Ias)
  Is7/3(I_0_s) -> Terminator6/1
  Is7/2(I_d_s) -> Display7/1
  Is7/1(I_q_s) -> Display6/1
  [angle] -> Is7/4(Angle)

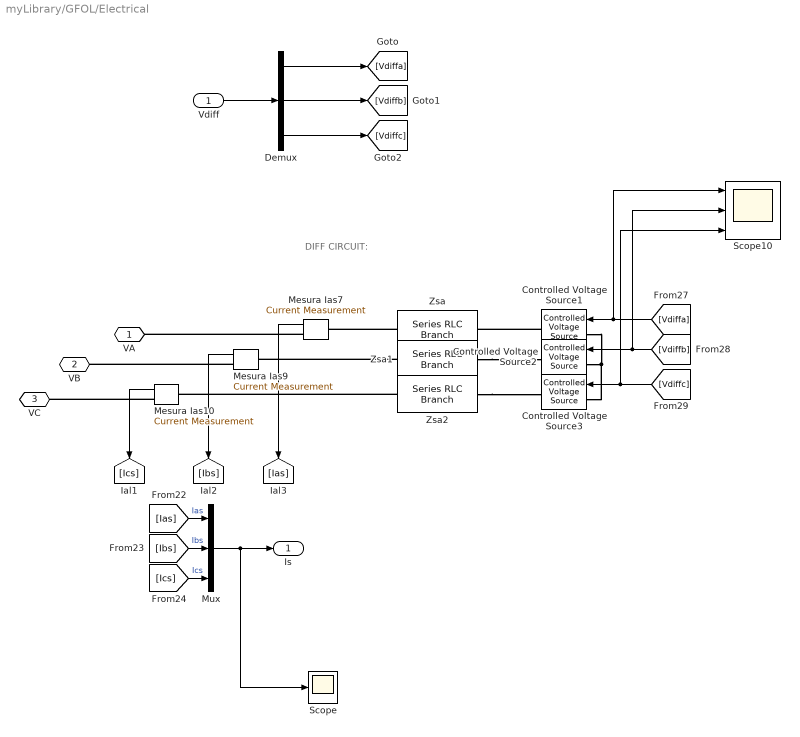
== system myLibrary/GFOL/Electrical ==
  note: DIFF CIRCUIT:
  Vdiff : Inport
  Controlled Voltage Source1 : spsControlledVoltageSourceLib/Controlled Voltage Source  Initialize=on  Source_Type=AC  Amplitude=initVSC.Udiff_mag  Phase=initVSC.angle_vdiff*180/pi  Frequency=T_VSC.fb  Measurements=None
  Controlled Voltage Source2 : spsControlledVoltageSourceLib/Controlled Voltage Source  Initialize=on  Source_Type=AC  Amplitude=initVSC.Udiff_mag  Phase=(initVSC.angle_vdiff -2*pi/3)*180/pi  Frequency=T_VSC.fb  Measurements=None
  Controlled Voltage Source3 : spsControlledVoltageSourceLib/Controlled Voltage Source  Initialize=on  Source_Type=AC  Amplitude=initVSC.Udiff_mag  Phase=(initVSC.angle_vdiff +2*pi/3)*180/pi  Frequency=T_VSC.fb  Measurements=None
  Demux : Demux  Outputs=3
  Mesura Ias10 : spsCurrentMeasurementLib/Current Measurement  PhasorSimulation=off  OutputType=Complex  PSBequivalent=0
  Mesura Ias7 : spsCurrentMeasurementLib/Current Measurement  PhasorSimulation=off  OutputType=Complex  PSBequivalent=0
  Mesura Ias9 : spsCurrentMeasurementLib/Current Measurement  PhasorSimulation=off  OutputType=Complex  PSBequivalent=0
  Mux : Mux  Inputs=3
  Scope : Scope
  Scope10 : Scope  NumInputPorts=3
  Zsa : spsSeriesRLCBranchLib/Series RLC Branch  LConnTagsString=__new0  RConnTagsString=__new0  BranchType=RL  Resistance=initVSC.Rc  Inductance=initVSC.Lc  SetiL0=off  InitialCurrent=initVSC.Isa  Capacitance=1e-6  Setx0=off  InitialVoltage=0  Measurements=None
  Zsa1 : spsSeriesRLCBranchLib/Series RLC Branch  LConnTagsString=__new0  RConnTagsString=__new0  BranchType=RL  Resistance=initVSC.Rc  Inductance=initVSC.Lc  SetiL0=on  InitialCurrent=initVSC.Isb  Capacitance=1e-6  Setx0=off  InitialVoltage=0  Measurements=None
  Zsa2 : spsSeriesRLCBranchLib/Series RLC Branch  LConnTagsString=__new0  RConnTagsString=__new0  BranchType=RL  Resistance=initVSC.Rc  Inductance=initVSC.Lc  SetiL0=on  InitialCurrent=initVSC.Isc  Capacitance=1e-6  Setx0=off  InitialVoltage=0  Measurements=None
  VA : PMIOPort  Side=Left
  VB : PMIOPort  Port=2  Side=Left
  VC : PMIOPort  Port=3  Side=Left
  Is : Outport
  wires:
  Mesura Ias10/1 -> [Ics]
  Mesura Ias7/1 -> [Ias]
  Mesura Ias9/1 -> [Ibs]
  Vdiff/1 -> Demux/1
  Demux/1 -> [Vdiffa]
  Demux/3 -> [Vdiffc]
  Demux/2 -> [Vdiffb]
  Mux/1 -> Scope/1, Is/1
  [Ics] -> Mux/3  "Ics"
  [Ibs] -> Mux/2  "Ibs"
  [Ias] -> Mux/1  "Ias"
  [Vdiffa] -> Controlled Voltage Source1/1, Scope10/1
  [Vdiffb] -> Scope10/2, Controlled Voltage Source2/1
  [Vdiffc] -> Controlled Voltage Source3/1, Scope10/3
  connections:
  Zsa1/LConn1 -- Controlled Voltage Source2/RConn1
  Mesura Ias7/RConn1 -- VA/RConn1
  Mesura Ias9/RConn1 -- VB/RConn1
  Mesura Ias10/RConn1 -- VC/RConn1
  Zsa/RConn1 -- Mesura Ias7/LConn1
  Zsa1/RConn1 -- Mesura Ias9/LConn1
  Zsa2/RConn1 -- Mesura Ias10/LConn1
  Controlled Voltage Source1/RConn1 -- Zsa/LConn1
  Zsa2/LConn1 -- Controlled Voltage Source3/RConn1
  Controlled Voltage Source3/LConn1 -- Controlled Voltage Source1/LConn1 -- Controlled Voltage Source2/LConn1

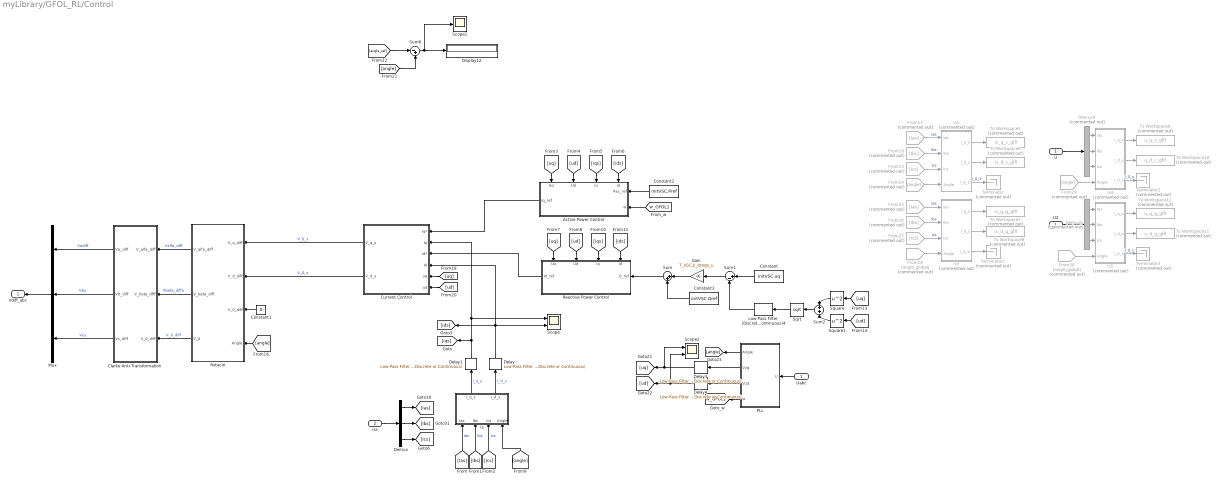
== system myLibrary/GFOL_RL/Control ==
  U : Inport
  Iss : Inport  Port=2
  Active Power Control : Subsystem
      settings: PortSchema="{\"entries\":[{\"content\":{\"sides\":[{\"content\":{\"connectorIds\":[\"In1\",\"In2\"]},\"type\":\"ConnectorPlacement.EquallySpacedRectSide\",\"uuid\":\"78fe08fc-97ab-4d3f-ad1e-a4935a540f0d\"},{\"content\":{\"connectorIds\":[\"Out1\"],\"side\":\"RIGHT\"},\"type\":\"ConnectorPlacement.EquallySpacedRectSide\",\"uuid\":\"fec6fd50-7083-47ad-a120-ce0b4b3eb939\"},{\"content\":{\"connectorIds\":[\"In3\",\"In4\",\"In5\",\"In6\"],\"side\":\"TOP\"},\"type\":\"ConnectorPlacement.EquallySpacedRectSide\",\"uuid\":\"cab1bf13-1988-4815-ae0e-163353411583\"}]},\"type\":\"ConnectorPlacement.EquallySpacedConnector\",\"uuid\":\"1108cbfd-0203-4acc-b5d3-05af7402b6e2\"}],\"packageUris\":[\"http://schema.mathworks.com/mf0/Connector/R2020b\"],\"version\":\"1.0\"}"
  Clarke Anti-Transformation : Subsystem
  Constant : Constant  Value=initVSC.uq
  Constant1 : Constant  Value=0
  Constant2 : Constant  Value=initVSC.Pref
  Constant3 : Constant  Value=initVSC.Qref
  Current Control : Subsystem
  Delay : eeGeneralControl/Low-Pass Filter (Discrete or Continuous)  K=1  T=init_VSC.delay  B=inf  A=-inf  init_option=Specify as parameter  x0=initVSC.idiffd  Ts=0
  Delay1 : eeGeneralControl/Low-Pass Filter (Discrete or Continuous)  K=1  T=init_VSC.delay  B=inf  A=-inf  init_option=Specify as parameter  x0=initVSC.idiffq  Ts=0
  Delay3 : eeGeneralControl/Low-Pass Filter (Discrete or Continuous)  K=1  T=init_VSC.delay  B=inf  A=-inf  init_option=Specify as parameter  x0=initVSC.uq  Ts=0
  Delay4 : eeGeneralControl/Low-Pass Filter (Discrete or Continuous)  K=1  T=init_VSC.delay  B=inf  A=-inf  init_option=Specify as parameter  x0=initVSC.ud  Ts=0
  Demux : Demux  Outputs=3
  Demux4 : Demux  Commented=on  Outputs=3
  Demux5 : Demux  Commented=on  Outputs=3
  Display12 : Display
  From17 : From  Commented=on  GotoTag=Ias
  From18 : From  Commented=on  GotoTag=Ibs
  From23 : From  Commented=on  GotoTag=Ics
  From24 : From  Commented=on  GotoTag=angle
  From25 : From  Commented=on  GotoTag=Ias
  From26 : From  Commented=on  GotoTag=Ibs
  From27 : From  Commented=on  GotoTag=Ics
  From28 : From  Commented=on  GotoTag=angle_global  TagVisibility=global
  From29 : From  Commented=on  GotoTag=angle
  From30 : From  Commented=on  GotoTag=angle_global  TagVisibility=global
  Gain : Gain  Gain=T_VSC.k_droop_u
  Is : Subsystem
  Is1 : Subsystem  Commented=on
  Is3 : Subsystem  Commented=on
  Is4 : Subsystem  Commented=on
  Is5 : Subsystem  Commented=on
  Low-Pass Filter (Discrete or Continuous)4 : eeGeneralControl/Low-Pass Filter (Discrete or Continuous)  K=1  T=T_VSC.tau_droop_u  B=inf  A=-inf  init_option=Specify as parameter  x0=initVSC.uq  Ts=-1
  Mux : Mux  Inputs=3
  PLL : Subsystem
  Reactive Power Control : Subsystem
      settings: PortSchema="{\"entries\":[{\"content\":{\"sides\":[{\"content\":{\"connectorIds\":[\"In1\"]},\"type\":\"ConnectorPlacement.EquallySpacedRectSide\",\"uuid\":\"78fe08fc-97ab-4d3f-ad1e-a4935a540f0d\"},{\"content\":{\"connectorIds\":[\"Out1\"],\"side\":\"RIGHT\"},\"type\":\"ConnectorPlacement.EquallySpacedRectSide\",\"uuid\":\"fec6fd50-7083-47ad-a120-ce0b4b3eb939\"},{\"content\":{\"connectorIds\":[\"In2\",\"In3\",\"In4\",\"In5\"],\"side\":\"TOP\"},\"type\":\"ConnectorPlacement.EquallySpacedRectSide\",\"uuid\":\"cab1bf13-1988-4815-ae0e-163353411583\"}]},\"type\":\"ConnectorPlacement.EquallySpacedConnector\",\"uuid\":\"1108cbfd-0203-4acc-b5d3-05af7402b6e2\"}],\"packageUris\":[\"http://schema.mathworks.com/mf0/Connector/R2020b\"],\"version\":\"1.0\"}"
  Rotació : Subsystem
  Scope : Scope  NumInputPorts=2
  Scope1 : Scope
  Scope2 : Scope  NumInputPorts=2
  Sqrt : Sqrt
  Square : Math  Operator=square
  Square1 : Math  Operator=square
  Sum : Sum  Inputs=|++
  Sum1 : Sum  Inputs=|+-
  Sum2 : Sum
  Sum6 : Sum  Inputs=|-+
  Terminator{,1..3} (4 alike) : Terminator  Commented=on
  To Workspace10 : ToWorkspace  Commented=on  VariableName=u_d_c_gfll  SampleTime=plots_step
  To Workspace11 : ToWorkspace  Commented=on  VariableName=u_d_g_gfll  SampleTime=plots_step
  To Workspace12 : ToWorkspace  Commented=on  VariableName=u_q_g_gfll  SampleTime=plots_step
  To Workspace5 : ToWorkspace  Commented=on  VariableName=is_q_c_gfll  SampleTime=plots_step
  To Workspace6 : ToWorkspace  Commented=on  VariableName=is_d_c_gfll  SampleTime=plots_step
  To Workspace7 : ToWorkspace  Commented=on  VariableName=is_q_g_gfll  SampleTime=plots_step
  To Workspace8 : ToWorkspace  Commented=on  VariableName=is_d_g_gfll  SampleTime=plots_step
  To Workspace9 : ToWorkspace  Commented=on  VariableName=u_q_c_gfll  SampleTime=plots_step
  U2 : InportShadow
  Uabc : InportShadow
  Vdiff_abc : Outport
  tag scope: w_GFOL1=global
  wires:
  Sqrt/1 -> Low-Pass Filter (Discrete or Continuous)4/1
  Delay4/1 -> [ud], Scope2/2
  Delay3/1 -> Scope2/1, [uq]
  Constant/1 -> Sum1/1
  Low-Pass Filter (Discrete or Continuous)4/1 -> Sum1/2
  Sum2/1 -> Sqrt/1
  Square1/1 -> Sum2/2
  Square/1 -> Sum2/1
  [ud] -> Square1/1
  [uq] -> Square/1
  Sum1/1 -> Gain/1
  Gain/1 -> Sum/1
  Constant3/1 -> Sum/2
  Sum/1 -> Reactive Power Control/1(Q_ref)
  [w_GFOL1] -> Active Power Control/2(w)
  PLL/4(w) -> [w_GFOL1]
  Is/2(I_d_s) -> Delay/1  "I_d_s"
  Is/1(I_q_s) -> Delay1/1  "I_q_s"
  [Ias] -> Is/1(Ias)  "Ias"
  [Ics] -> Is/3(Ics)  "Ics"
  [Ibs] -> Is/2(Ibs)  "Ibs"
  PLL/1(Angle) -> [angle]
  Uabc/1 -> PLL/1(U)
  Demux/1 -> [Ias]
  Demux/2 -> [Ibs]
  Demux/3 -> [Ics]
  Iss/1 -> Demux/1
  [angle] -> Is/4(Angle)
  [angle] -> Rotació/4(Angle)
  Current Control/1(V_q_s) -> Rotació/1(V_q_diff)  "V_0_s"
  Current Control/2(V_d_s) -> Rotació/2(V_d_diff)  "V_0_s"
  [uq] -> Current Control/5(uq)
  [ud] -> Current Control/6(ud)
  [angle] -> Sum6/2
  Sum6/1 -> Scope1/1, Display12/1
  [angle_ref] -> Sum6/1
  From17/1 -> Is1/1(Ias)  "Ias"
  From18/1 -> Is1/2(Ibs)  "Ibs"
  From23/1 -> Is1/3(Ics)  "Ics"
  From24/1 -> Is1/4(Angle)
  From27/1 -> Is3/3(Ics)  "Ics"
  From26/1 -> Is3/2(Ibs)  "Ibs"
  From25/1 -> Is3/1(Ias)  "Ias"
  From28/1 -> Is3/4(Angle)
  U/1 -> Demux4/1
  Demux4/1 -> Is4/1(Ias)
  Demux4/2 -> Is4/2(Ibs)
  Demux4/3 -> Is4/3(Ics)
  From29/1 -> Is4/4(Angle)
  From30/1 -> Is5/4(Angle)
  Demux5/3 -> Is5/3(Ics)
  Demux5/2 -> Is5/2(Ibs)
  Demux5/1 -> Is5/1(Ias)
  U2/1 -> Demux5/1
  Is1/1(I_q_s) -> To Workspace5/1
  Is1/2(I_d_s) -> To Workspace6/1
  Is3/1(I_q_s) -> To Workspace7/1
  Is3/2(I_d_s) -> To Workspace8/1
  Is4/1(I_q_s) -> To Workspace9/1
  Is4/2(I_d_s) -> To Workspace10/1
  Is5/1(I_q_s) -> To Workspace12/1
  Is5/2(I_d_s) -> To Workspace11/1
  Is1/3(I_0_s) -> Terminator/1  "I_0_s"
  Is3/3(I_0_s) -> Terminator1/1
  Is4/3(I_0_s) -> Terminator2/1  "I_0_s"
  Is5/3(I_0_s) -> Terminator3/1  "I_0_s"
  Rotació/1(V_alfa_diff) -> Clarke Anti-Transformation/1(V_alfa_diff)  "Valfa_diff"
  Rotació/2(V_beta_diff) -> Clarke Anti-Transformation/2(V_beta_dfff)  "Vbeta_diffa"
  Clarke Anti-Transformation/1(Va_diff) -> Mux/1  "Vadiff"
  Rotació/3(V_0) -> Clarke Anti-Transformation/3(V_0_diff)  "V_0_diff"
  Clarke Anti-Transformation/3(Vc_diff) -> Mux/3  "Vcu"
  Clarke Anti-Transformation/2(Vb_diff) -> Mux/2  "Vbu"
  Mux/1 -> Vdiff_abc/1
  [uq] -> Active Power Control/6(Uq)
  [ud] -> Active Power Control/5(Ud)
  Active Power Control/1(Iq_ref) -> Current Control/1(Iq*)
  Delay/1 -> Scope/2, Current Control/4(Id), [ids]
  Delay1/1 -> Current Control/2(Iq), Scope/1, [iqs]
  Constant1/1 -> Rotació/3(V_0_diff)
  PLL/2(Vzq) -> Delay3/1
  PLL/3(Vzd) -> Delay4/1
  [iqs] -> Active Power Control/4(iq)
  [ids] -> Active Power Control/3(id)
  Constant2/1 -> Active Power Control/1(Pac_ref)
  [ids] -> Reactive Power Control/2(id)
  [iqs] -> Reactive Power Control/3(iq)
  [ud] -> Reactive Power Control/4(Ud)
  [uq] -> Reactive Power Control/5(Uq)
  Reactive Power Control/1(Id_ref) -> Current Control/3(Id*)

== system myLibrary/GFOL_RL/Electrical ==
  note: DIFF CIRCUIT:
  Vdiff : Inport
  Controlled Voltage Source1 : spsControlledVoltageSourceLib/Controlled Voltage Source  Initialize=on  Source_Type=AC  Amplitude=initVSC.Udiff_mag  Phase=initVSC.angle_vdiff*180/pi  Frequency=T_VSC.fb  Measurements=None
  Controlled Voltage Source2 : spsControlledVoltageSourceLib/Controlled Voltage Source  Initialize=on  Source_Type=AC  Amplitude=initVSC.Udiff_mag  Phase=(initVSC.angle_vdiff -2*pi/3)*180/pi  Frequency=T_VSC.fb  Measurements=None
  Controlled Voltage Source3 : spsControlledVoltageSourceLib/Controlled Voltage Source  Initialize=on  Source_Type=AC  Amplitude=initVSC.Udiff_mag  Phase=(initVSC.angle_vdiff +2*pi/3)*180/pi  Frequency=T_VSC.fb  Measurements=None
  Demux : Demux  Outputs=3
  Mesura Ias10 : spsCurrentMeasurementLib/Current Measurement  PhasorSimulation=off  OutputType=Complex  PSBequivalent=0
  Mesura Ias7 : spsCurrentMeasurementLib/Current Measurement  PhasorSimulation=off  OutputType=Complex  PSBequivalent=0
  Mesura Ias9 : spsCurrentMeasurementLib/Current Measurement  PhasorSimulation=off  OutputType=Complex  PSBequivalent=0
  Mux : Mux  Inputs=3
  Scope : Scope
  Scope10 : Scope  NumInputPorts=3
  Zsa : spsSeriesRLCBranchLib/Series RLC Branch  LConnTagsString=__new0  RConnTagsString=__new0  BranchType=RL  Resistance=initVSC.Rc  Inductance=initVSC.Lc  SetiL0=off  InitialCurrent=initVSC.Isa  Capacitance=1e-6  Setx0=off  InitialVoltage=0  Measurements=None
  Zsa1 : spsSeriesRLCBranchLib/Series RLC Branch  LConnTagsString=__new0  RConnTagsString=__new0  BranchType=RL  Resistance=initVSC.Rc  Inductance=initVSC.Lc  SetiL0=on  InitialCurrent=initVSC.Isb  Capacitance=1e-6  Setx0=off  InitialVoltage=0  Measurements=None
  Zsa2 : spsSeriesRLCBranchLib/Series RLC Branch  LConnTagsString=__new0  RConnTagsString=__new0  BranchType=RL  Resistance=initVSC.Rc  Inductance=initVSC.Lc  SetiL0=on  InitialCurrent=initVSC.Isc  Capacitance=1e-6  Setx0=off  InitialVoltage=0  Measurements=None
  VA : PMIOPort  Side=Left
  VB : PMIOPort  Port=2  Side=Left
  VC : PMIOPort  Port=3  Side=Left
  Is : Outport
  wires:
  Mesura Ias10/1 -> [Ics]
  Mesura Ias7/1 -> [Ias]
  Mesura Ias9/1 -> [Ibs]
  Vdiff/1 -> Demux/1
  Demux/1 -> [Vdiffa]
  Demux/3 -> [Vdiffc]
  Demux/2 -> [Vdiffb]
  Mux/1 -> Scope/1, Is/1
  [Ics] -> Mux/3  "Ics"
  [Ibs] -> Mux/2  "Ibs"
  [Ias] -> Mux/1  "Ias"
  [Vdiffa] -> Controlled Voltage Source1/1, Scope10/1
  [Vdiffb] -> Scope10/2, Controlled Voltage Source2/1
  [Vdiffc] -> Controlled Voltage Source3/1, Scope10/3
  connections:
  Zsa1/LConn1 -- Controlled Voltage Source2/RConn1
  Mesura Ias7/RConn1 -- VA/RConn1
  Mesura Ias9/RConn1 -- VB/RConn1
  Mesura Ias10/RConn1 -- VC/RConn1
  Zsa/RConn1 -- Mesura Ias7/LConn1
  Zsa1/RConn1 -- Mesura Ias9/LConn1
  Zsa2/RConn1 -- Mesura Ias10/LConn1
  Controlled Voltage Source1/RConn1 -- Zsa/LConn1
  Zsa2/LConn1 -- Controlled Voltage Source3/RConn1
  Controlled Voltage Source3/LConn1 -- Controlled Voltage Source1/LConn1 -- Controlled Voltage Source2/LConn1
